simulink model "crane_model"  (R2025b)
settings: Solver=ode4  StartTime=0.0  StopTime=10  FixedStep=0.001  RelTol=1e-3
values from neighbouring files (symbols this model uses):
  F_max = P/v    (= 900)    [crane_data.m]
  l = 1.5    [crane_data.m]
  M = 250    [crane_data.m]
  m_hook_and_payload = m_hook+m_payload    (= 25)    [crane_data.m]
settings Model: Creator=maliha  LastModifiedBy=maliha

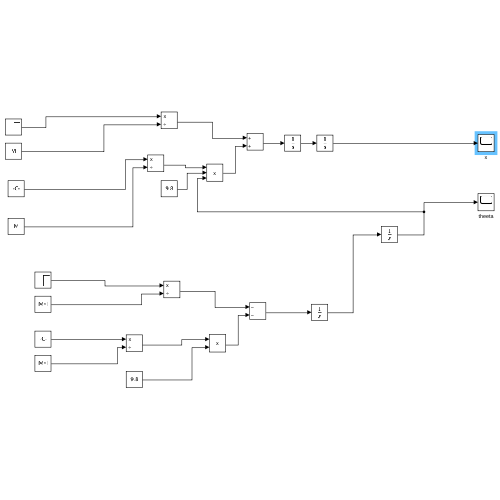
[thumbnail: Simulink's stored preview of the top-level diagram]
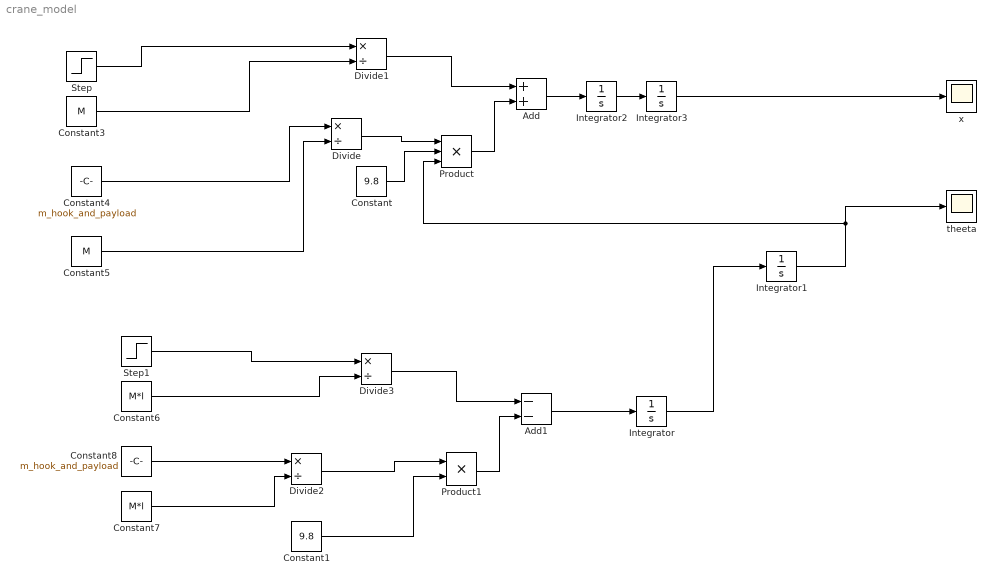
== system crane_model ==
  Add : Sum
  Add1 : Sum  Inputs=--
  Constant : Constant  Value=9.8
  Constant1 : Constant  Value=9.8
  Constant3 : Constant  Value=M
  Constant4 : Constant  Value=m_hook_and_payload
  Constant5 : Constant  Value=M
  Constant6 : Constant  Value=M*l
  Constant7 : Constant  Value=M*l
  Constant8 : Constant  Value=m_hook_and_payload
  Divide{,1..3} (4 alike) : Product  Inputs=*/
  Integrator{,1..3} (4 alike) : Integrator
  Product : Product  Inputs=3
  Product1 : Product
  Step : Step  Time=F_max  SampleTime=0
  Step1 : Step  Time=F_max  SampleTime=0
  theeta : Scope
      settings: ActiveDisplayYMinimum=-36.749999999996128  ActiveDisplayYMaximum=4.0833333333329023
  x : Scope
      settings: ActiveDisplayYMinimum=-301.79742907799982  ActiveDisplayYMaximum=48.348404255316893
  wires:
  Step/1 -> Divide1/1
  Product/1 -> Add/2
  Divide/1 -> Product/1
  Constant4/1 -> Divide/1
  Constant5/1 -> Divide/2
  Constant/1 -> Product/2
  Divide1/1 -> Add/1
  Constant3/1 -> Divide1/2
  Constant1/1 -> Product1/2
  Product1/1 -> Add1/2
  Add1/1 -> Integrator/1
  Divide3/1 -> Add1/1
  Constant6/1 -> Divide3/2
  Step1/1 -> Divide3/1
  Constant8/1 -> Divide2/1
  Constant7/1 -> Divide2/2
  Divide2/1 -> Product1/1
  Integrator/1 -> Integrator1/1
  Add/1 -> Integrator2/1
  Integrator2/1 -> Integrator3/1
  Integrator3/1 -> x/1
  Integrator1/1 -> Product/3, theeta/1
